simulink model "adrc_eso3"  (Simulink 7.9)
settings: Solver=ode45  StartTime=0.0  StopTime=10  RelTol=1e-3
undefined symbols (not defined in the file): a0, a1, b, wc, wo
settings Model: Creator=jasontatsumi  LastModifiedBy=Gao
settings DebuggingCC: FcnCallInpInsideContextMsg=Use local settings
settings GRTTargetCC: CombineOutputUpdateFcns=off  GRTInterface=on

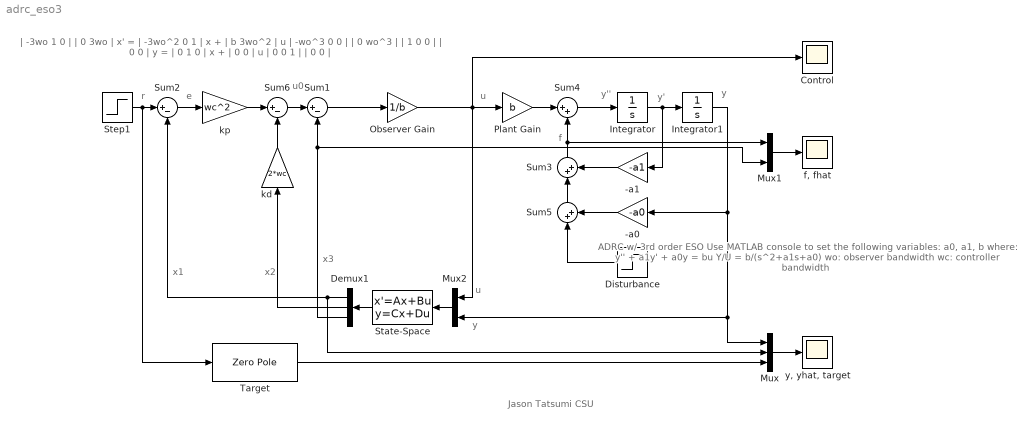
== system adrc_eso3 ==
  note: y'
  note: y''
  note: f
  note: u
  note: u0
  note: y
  note: u
  note: x1
  note: x3
  note: ADRC w/ 3rd order ESO
      |
      | Use MATLAB console
      | to set the following
      | variables:
      |
      | a0, a1,  b where:
      | y'' + a1y' + a0y = bu
      | Y/U = b/(s^2+a1s+a0)
      |
      | wo: observer bandwidth
      | wc: controller bandwidth
  note: | -3wo   1 0 |     | 0 3wo   |
      | x' = | -3wo^2 0 1 | x + | b 3wo^2 | u
      |      | -wo^3  0 0 |     | 0 wo^3  |
      |
      |      | 1 0 0 |     | 0 0 |
      | y  = | 0 1 0 | x + | 0 0 | u
      |      | 0 0 1 |     | 0 0 |
  note: e
  note: r
  note: x2
  note: y
  note: Jason Tatsumi
      | CSU
  -a0 : Gain  Gain=-a0
  -a1 : Gain  Gain=-a1
  Control : Scope
      settings: TimeRange=10  YMin=0  YMax=1
  Demux1 : Demux  Outputs=3
  Disturbance : Step  Time=6  After=50  SampleTime=0
  Integrator : Integrator
  Integrator1 : Integrator
  Mux : Mux  Inputs=3
  Mux1 : Mux  Inputs=2
  Mux2 : Mux  Inputs=2
  Observer Gain : Gain  Gain=1/b
  Plant Gain : Gain  Gain=b
  State-Space : StateSpace  A=[-3*wo 1 0;-3*wo^2 0 1;-wo^3 0 0]  B=[0 3*wo;b 3*wo^2 ; 0 wo^3 ]  C=eye(3)  D=zeros(3,2)
  Step1 : Step  SampleTime=0
  Sum1 : Sum  Inputs=|+-
  Sum2 : Sum  Inputs=|+-
  Sum3 : Sum  Inputs=|++
  Sum4 : Sum  Inputs=|++
  Sum5 : Sum  Inputs=|++
  Sum6 : Sum  Inputs=|+-
  Target : ZeroPole  Zeros=[]  Poles=[-wc -wc]  Gain=[wc^2]
  "f, fhat" : Scope
      settings: TimeRange=10  YMin=0  YMax=1  SaveName=ScopeData2
  kd : Gain  Gain=2*wc
  kp : Gain  Gain=wc^2
  "y, yhat, target" : Scope
      settings: TimeRange=10  YMin=0  YMax=1
  wires:
  Sum1/1 -> Observer Gain/1
  Sum2/1 -> kp/1
  Step1/1 -> Sum2/1, Target/1
  Sum4/1 -> Integrator/1
  Observer Gain/1 -> Mux2/1, Control/1, Plant Gain/1
  Demux1/1 -> Sum2/2, Mux/2
  -a1/1 -> Sum3/2
  Disturbance/1 -> Sum5/1
  Plant Gain/1 -> Sum4/1
  Sum3/1 -> Sum4/2, Mux1/1
  Mux/1 -> "y, yhat, target"/1
  Mux1/1 -> "f, fhat"/1
  Target/1 -> Mux/3
  Integrator1/1 -> -a0/1, Mux2/2, Mux/1
  -a0/1 -> Sum5/2
  Sum5/1 -> Sum3/1
  Mux2/1 -> State-Space/1
  State-Space/1 -> Demux1/1
  Sum6/1 -> Sum1/1
  kp/1 -> Sum6/1
  kd/1 -> Sum6/2
  Demux1/3 -> Sum1/2, Mux1/2
  Demux1/2 -> kd/1
  Integrator/1 -> Integrator1/1, -a1/1
